simulink model "progetto_ese1_sim_easy"  (R2024a)
settings: Solver=VariableStepAuto  StartTime=0.0  StopTime=10.0  RelTol=1e-3
values from neighbouring files (symbols this model uses):
  g = 9.81    [progetto_ese1_primo.m]
  m = 1.4    [progetto_ese1_primo.m]
undefined symbols (not defined in the file or in its folder): phi, psi, theta, U1
settings Model: Creator=USER  LastModifiedBy=USER

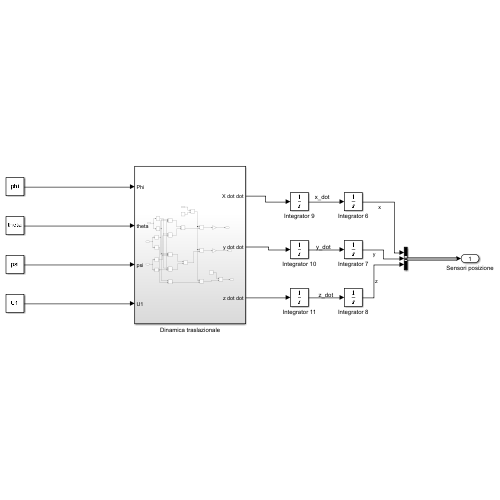
[thumbnail: Simulink's stored preview of the top-level diagram]
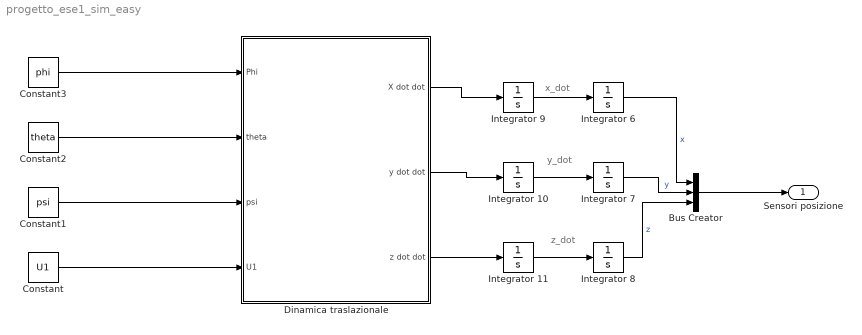
== system progetto_ese1_sim_easy ==
  note: z_dot
  note: x_dot
  note: y_dot
  Bus Creator : BusCreator  Inputs=3
  Constant : Constant  Value=U1
  Constant1 : Constant  Value=psi
  Constant2 : Constant  Value=theta
  Constant3 : Constant  Value=phi
  Dinamica traslazionale : Subsystem
  Integrator 10 : Integrator
  Integrator 11 : Integrator
  Integrator 6 : Integrator  ContinuousStateAttributes='X_out'
  Integrator 7 : Integrator  ContinuousStateAttributes='Y_out'
  Integrator 8 : Integrator  ContinuousStateAttributes='Z_out'
  Integrator 9 : Integrator
  Sensori posizione : Outport
  wires:
  Dinamica traslazionale/2(y dot dot) -> Integrator 10/1
  Integrator 11/1 -> Integrator 8/1
  Integrator 8/1 -> Bus Creator/3  "z"
  Dinamica traslazionale/3(z dot dot) -> Integrator 11/1
  Integrator 6/1 -> Bus Creator/1  "x"
  Dinamica traslazionale/1(X dot dot) -> Integrator 9/1
  Integrator 7/1 -> Bus Creator/2  "y"
  Integrator 9/1 -> Integrator 6/1
  Integrator 10/1 -> Integrator 7/1
  Bus Creator/1 -> Sensori posizione/1
  Constant3/1 -> Dinamica traslazionale/1(Phi)
  Constant2/1 -> Dinamica traslazionale/2(theta)
  Constant1/1 -> Dinamica traslazionale/3(psi)
  Constant/1 -> Dinamica traslazionale/4(U1)

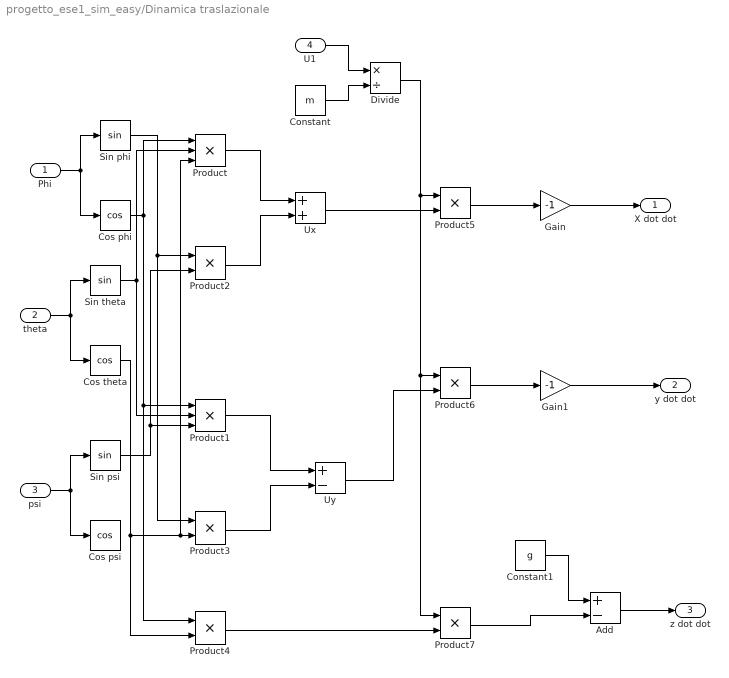
== system progetto_ese1_sim_easy/Dinamica traslazionale ==
  Phi : Inport
  theta : Inport  Port=2
  psi : Inport  Port=3
  U1 : Inport  Port=4
  Add : Sum  Inputs=+-
  Constant : Constant  Value=m
  Constant1 : Constant  Value=g
  Cos phi : Trigonometry  Operator=cos
  Cos psi : Trigonometry  Operator=cos
  Cos theta : Trigonometry  Operator=cos
  Divide : Product  Inputs=*/
  Gain : Gain  Gain=-1
  Gain1 : Gain  Gain=-1
  Product : Product  Inputs=3
  Product1 : Product  Inputs=3
  Product{2..7} (6 alike) : Product
  Sin phi : Trigonometry
  Sin psi : Trigonometry
  Sin theta : Trigonometry
  Ux : Sum
  Uy : Sum  Inputs=+-
  X dot dot : Outport
  y dot dot : Outport  Port=2
  z dot dot : Outport  Port=3
  wires:
  Phi/1 -> Cos phi/1, Sin phi/1
  theta/1 -> Cos theta/1, Sin theta/1
  psi/1 -> Cos psi/1, Sin psi/1
  Sin phi/1 -> Product2/1, Product3/1
  Cos phi/1 -> Product1/1, Product4/1, Product/1
  Sin theta/1 -> Product1/2, Product/2
  Cos theta/1 -> Product/3, Product3/2, Product4/2
  Sin psi/1 -> Product1/3, Product2/2
  Product/1 -> Ux/1
  Product2/1 -> Ux/2
  Product1/1 -> Uy/1
  Product3/1 -> Uy/2
  Ux/1 -> Product5/2
  Product4/1 -> Product7/2
  Uy/1 -> Product6/2
  Constant/1 -> Divide/2
  U1/1 -> Divide/1
  Divide/1 -> Product7/1, Product6/1, Product5/1
  Product6/1 -> Gain1/1
  Product5/1 -> Gain/1
  Gain/1 -> X dot dot/1
  Gain1/1 -> y dot dot/1
  Product7/1 -> Add/2
  Constant1/1 -> Add/1
  Add/1 -> z dot dot/1
